simulink model "eightrep"  (R2020a)
settings: Solver=VariableStepAuto  StartTime=0.0  StopTime=10.0  RelTol=1e-3
undefined symbols (not defined in the file): d, J, Kd, Ki, Kp, sigbuilder_block
settings Model: Creator=Admin  LastModifiedBy=Admin

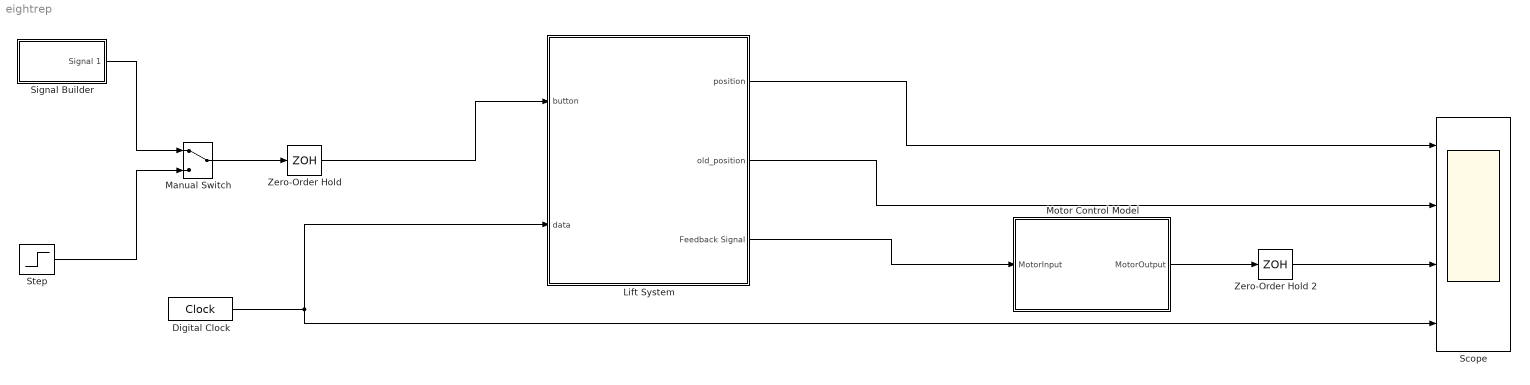
== system eightrep ==
  "Digital Clock " : DigitalClock
  Lift System : Subsystem
  "Manual Switch " : ManualSwitch
  Motor Control Model : Subsystem
  Scope : Scope  NumInputPorts=4
  Signal Builder : Subsystem  Tag=STV Subsys  LoadFcn=sigbuilder_block('load');  StartFcn=sigbuilder_block('start');  StopFcn=sigbuilder_block('stop');  ClipboardFcn=sigbuilder_block('clipboard');  mask(Sigbuilder block){tuvar=[0:10]}
      mask help: Simulink:masks:SigbuilderBlock_MD
      mask init:
      | if ~strcmp(get_param(bdroot(gcbh),'SimulationStatus'),'stopped') tuvar = sigbuilder_block('maskInit'); end
      settings: CopyFcn=sigbuilder_block('copy');  DeleteFcn=sigbuilder_block('delete');  ModelCloseFcn=sigbuilder_block('modelClose');  PreSaveFcn=sigbuilder_block('preSave');  PauseFcn=sigbuilder_block('pause');  ContinueFcn=sigbuilder_block('continue');  NameChangeFcn=sigbuilder_block('namechange');  OpenFcn=sigbuilder_block('open',[437.6 199.2 550.4 400 ]);  CloseFcn=sigbuilder_block('close');
      mask Display: plot(0, 0, 100, 100,[2, 2, 32, 32, 2], [68, 8, 8, 68, 68],[32, 2], [38, 38], [32, 19, 2],[53, 60, 44], [32, 17, 17, 2],[16, 16, 31, 31]);txt = getActiveGroup(gcbh);text(2, 100, txt,'verticalAlignment', 'top');
  Step : Step  SampleTime=0
  "Zero-Order Hold " : ZeroOrderHold  SampleTime=-1
  Zero-Order Hold 2 : ZeroOrderHold  SampleTime=-1
  wires:
  Step/1 -> "Manual Switch "/2
  "Manual Switch "/1 -> "Zero-Order Hold "/1
  Signal Builder/1(Signal 1) -> "Manual Switch "/1
  Motor Control Model/1(MotorOutput) -> Zero-Order Hold 2/1
  Zero-Order Hold 2/1 -> Scope/3
  "Digital Clock "/1 -> Lift System/2(data), Scope/4
  "Zero-Order Hold "/1 -> Lift System/1(button)
  Lift System/1(position) -> Scope/1
  Lift System/2(old_position) -> Scope/2
  Lift System/3(Feedback Signal) -> Motor Control Model/1(MotorInput)

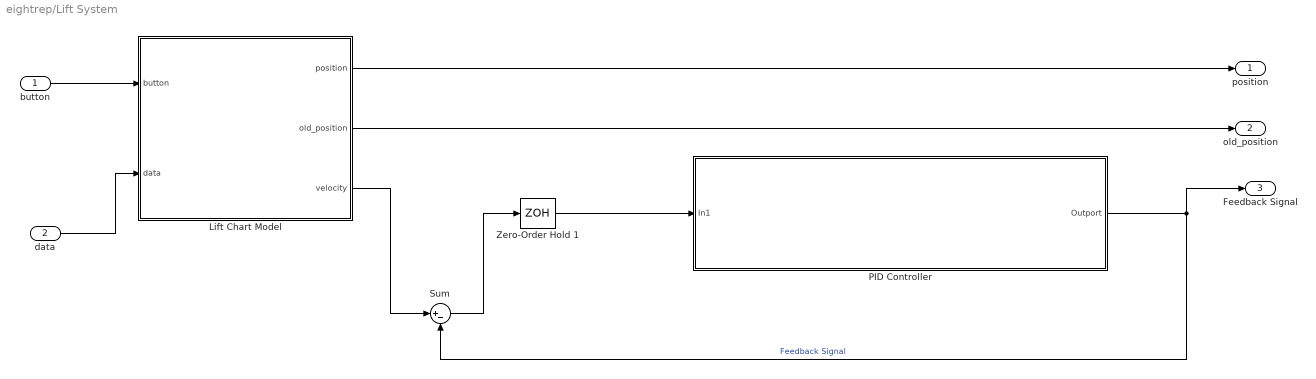
== system eightrep/Lift System ==
  button : Inport
  data : Inport  Port=2
  Lift Chart Model : Stateflow chart  TreatAsAtomicUnit=on
  "PID Controller " : Subsystem
  Sum : Sum  Inputs=|+-
  Zero-Order Hold 1 : ZeroOrderHold  SampleTime=-1
  position : Outport
  old_position : Outport  Port=2
  Feedback Signal : Outport  Port=3
  wires:
  "PID Controller "/1(Outport) -> Sum/2, Feedback Signal/1  "Feedback Signal"
  data/1 -> Lift Chart Model/2(data)
  Zero-Order Hold 1/1 -> "PID Controller "/1(In1)
  Sum/1 -> Zero-Order Hold 1/1
  Lift Chart Model/3(velocity) -> Sum/1
  button/1 -> Lift Chart Model/1(button)
  Lift Chart Model/1(position) -> position/1
  Lift Chart Model/2(old_position) -> old_position/1

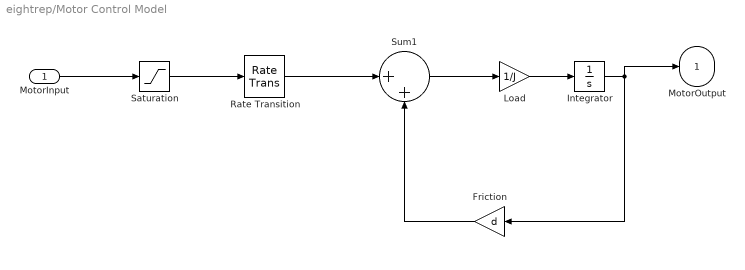
== system eightrep/Motor Control Model ==
  MotorInput : Inport
  Friction : Gain  Gain=d
  Integrator : Integrator
  Load : Gain  Gain=1/J
  "Rate Transition " : RateTransition
  "Saturation " : Saturate
  Sum1 : Sum  Inputs=|++
  MotorOutput : Outport
  wires:
  MotorInput/1 -> "Saturation "/1
  "Saturation "/1 -> "Rate Transition "/1
  "Rate Transition "/1 -> Sum1/1
  Sum1/1 -> Load/1
  Load/1 -> Integrator/1
  Friction/1 -> Sum1/2
  Integrator/1 -> MotorOutput/1, Friction/1

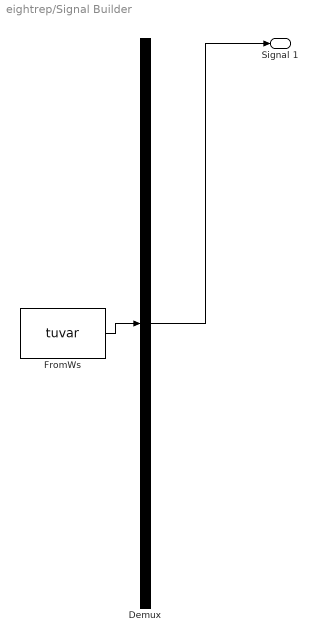
== system eightrep/Signal Builder ==
  Demux : Demux  Tag=STV Demux  Outputs=1
      settings: DisplayOption=none
  FromWs : FromWorkspace  Tag=STV FromWs  VariableName=tuvar
      SigBuilderData=|
      | common.afterFinalStr = 'Extrapolate'
      | common.sampleTime = 0
      | dataSet.timeRange = [0 10]
      | dataSet.name = 'Group 1'
      | sbobj.Groups.Name = 'Group 1'
      | sbobj.Groups.Signals.Name = 'Signal 1'
      | sbobj.Groups.Signals.XData = [0 4 4 6 6 10]
      | sbobj.Groups.Signals.YData = [0 0 1 1 0 0]
  Signal 1 : Outport  Tag=STV Outport
  wires:
  Demux/1 -> Signal 1/1
  FromWs/1 -> Demux/1

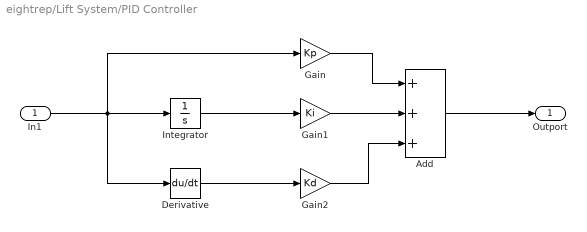
== system eightrep/Lift System/PID Controller  ==
  In1 : Inport
  Add : Sum  Inputs=+++
  Derivative : Derivative
  Gain : Gain  Gain=Kp
  Gain1 : Gain  Gain=Ki
  Gain2 : Gain  Gain=Kd
  Integrator : Integrator
  Outport : Outport
  wires:
  Add/1 -> Outport/1
  In1/1 -> Gain/1, Derivative/1, Integrator/1
  Gain1/1 -> Add/2
  Gain/1 -> Add/1
  Derivative/1 -> Gain2/1
  Integrator/1 -> Gain1/1
  Gain2/1 -> Add/3

== stateflow chart eightrep/Lift System/Lift Chart Model ==
  note: 1)If on 5th floor and button is less than zero
      | 2)or if on ground floor and button is more than zero
      | 3)Run Lift
  note: 1)Run lift motor if button has been pushed
  state ReadInput
  state Motor
    entry:
    position=velocity*t+old_position
    exit:
    old_position =position;
    velocity=button;
  state ReadInput2
  note: 1)If on 5th floor and button is more than zero
      | 2)or if on ground floor and button is less than zero
      | 3) Stope Lift
  state Hold
  state Stop
    entry:
    velocity=0;
  Motor -> ReadInput [order 3] : [(button>0&&position<5)||(button<0&&position>0)]
  ReadInput -> Motor [order 2]
  Hold -> ReadInput [order 2] : [button>0&&position<3]
  ReadInput -> Hold [order 1] : [[(button>0&&position>5)||(button<0&&position<0)]]
  ReadInput2 -> Motor : [(button>0&&position<5)||(button<0&&position>0)]
  Motor -> ReadInput2 [order 2]
  Motor -> Stop [order 1] : [position>5||position<0]
  Hold -> ReadInput2 [order 3] : [button>0&&position>0]
  Hold -> Stop [order 1]
  Stop -> Hold
  (default) -> Hold
  data: button input; position output; old_position output; velocity output; data input
